simulink model "Sensor_Implementation"  (R2017a)
settings: Solver=VariableStepAuto  StartTime=0.0  StopTime=1000  RelTol=1e-3
libraries: simulink x6
settings Model: Creator=GusBus  LastModifiedBy=GusBus

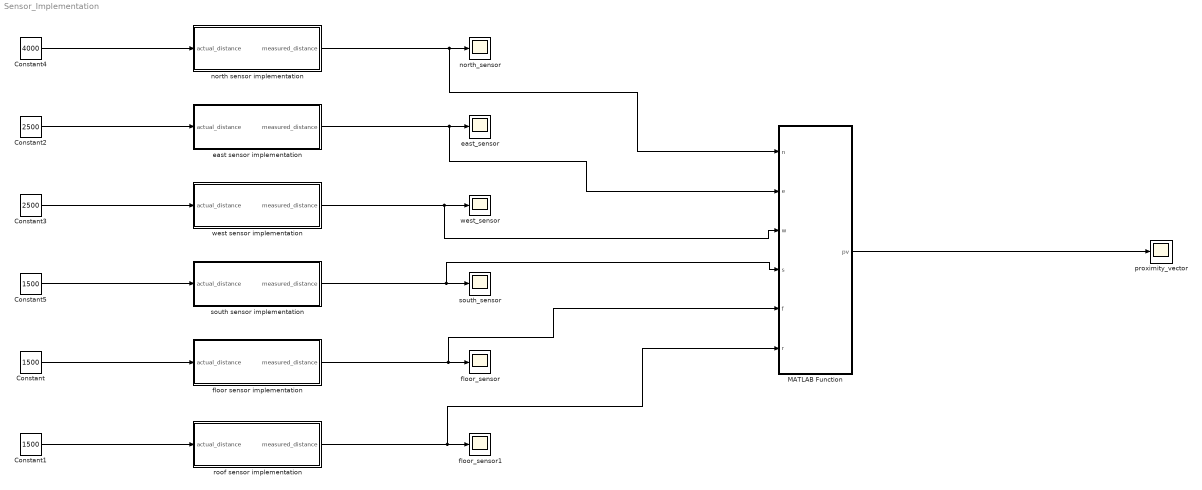
== system Sensor_Implementation ==
  Constant : Constant  Value=1500
  Constant1 : Constant  Value=1500
  Constant2 : Constant  Value=2500
  Constant3 : Constant  Value=2500
  Constant4 : Constant  Value=4000
  Constant5 : Constant  Value=1500
  MATLAB Function : MATLAB Function  TreatAsAtomicUnit=on
  east sensor implementation : Subsystem
  east_sensor : Scope
  floor sensor implementation : Subsystem
  floor_sensor : Scope
  floor_sensor1 : Scope
  north sensor implementation : Subsystem
  north_sensor : Scope
  proximity_vector : Scope
  roof sensor implementation : Subsystem
  south sensor implementation : Subsystem
  south_sensor : Scope
  west sensor implementation : Subsystem
  west_sensor : Scope
  wires:
  Constant/1 -> floor sensor implementation/1(actual_distance)
  floor sensor implementation/1(measured_distance) -> MATLAB Function/5(f), floor_sensor/1
  roof sensor implementation/1(measured_distance) -> MATLAB Function/6(r), floor_sensor1/1
  Constant1/1 -> roof sensor implementation/1(actual_distance)
  east sensor implementation/1(measured_distance) -> east_sensor/1, MATLAB Function/2(e)
  Constant2/1 -> east sensor implementation/1(actual_distance)
  west sensor implementation/1(measured_distance) -> MATLAB Function/3(w), west_sensor/1
  Constant3/1 -> west sensor implementation/1(actual_distance)
  Constant4/1 -> north sensor implementation/1(actual_distance)
  north sensor implementation/1(measured_distance) -> MATLAB Function/1(n), north_sensor/1
  Constant5/1 -> south sensor implementation/1(actual_distance)
  south sensor implementation/1(measured_distance) -> MATLAB Function/4(s), south_sensor/1
  MATLAB Function/1(pv) -> proximity_vector/1

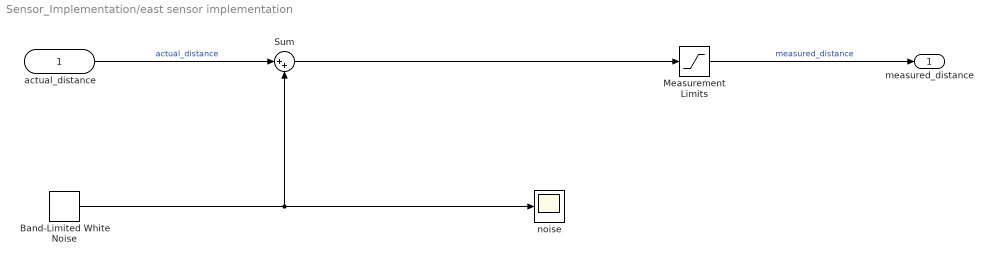
== system Sensor_Implementation/east sensor implementation ==
  actual_distance : Inport
  Band-Limited White Noise : simulink/Sources/Band-Limited White Noise  Cov=[0.01]  Ts=0.1  seed=[23341]
  Measurement Limits : Saturate  UpperLimit=4000  LowerLimit=40
  Sum : Sum  Inputs=|++
  noise : Scope
  measured_distance : Outport
  wires:
  actual_distance/1 -> Sum/1  "actual_distance"
  Measurement Limits/1 -> measured_distance/1  "measured_distance"
  Band-Limited White Noise/1 -> noise/1, Sum/2
  Sum/1 -> Measurement Limits/1

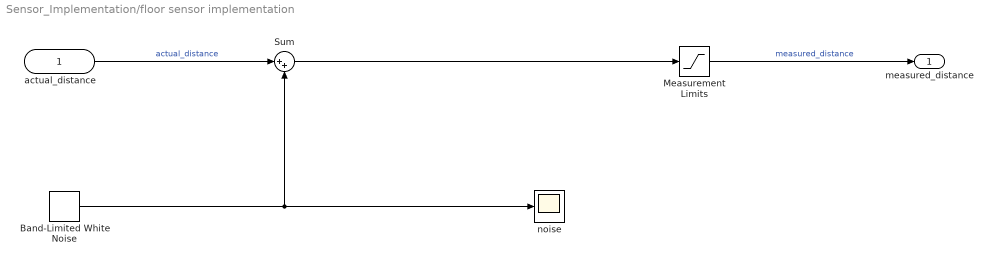
== system Sensor_Implementation/floor sensor implementation ==
  actual_distance : Inport
  Band-Limited White Noise : simulink/Sources/Band-Limited White Noise  Cov=[0.01]  Ts=0.1  seed=[23341]
  Measurement Limits : Saturate  UpperLimit=4000  LowerLimit=40
  Sum : Sum  Inputs=|++
  noise : Scope
  measured_distance : Outport
  wires:
  actual_distance/1 -> Sum/1  "actual_distance"
  Measurement Limits/1 -> measured_distance/1  "measured_distance"
  Band-Limited White Noise/1 -> noise/1, Sum/2
  Sum/1 -> Measurement Limits/1

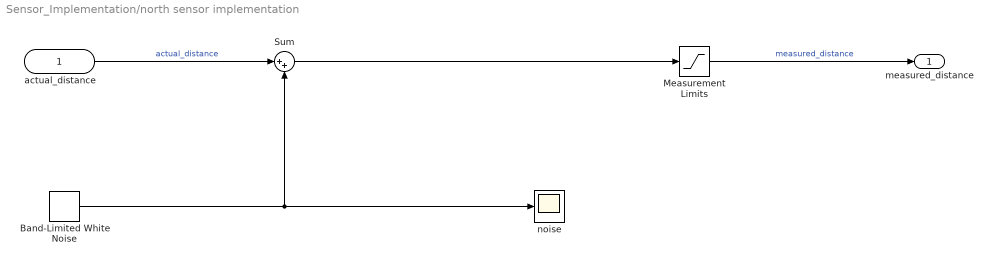
== system Sensor_Implementation/north sensor implementation ==
  actual_distance : Inport
  Band-Limited White Noise : simulink/Sources/Band-Limited White Noise  Cov=[0.01]  Ts=0.1  seed=[23341]
  Measurement Limits : Saturate  UpperLimit=4000  LowerLimit=40
  Sum : Sum  Inputs=|++
  noise : Scope
  measured_distance : Outport
  wires:
  actual_distance/1 -> Sum/1  "actual_distance"
  Measurement Limits/1 -> measured_distance/1  "measured_distance"
  Band-Limited White Noise/1 -> noise/1, Sum/2
  Sum/1 -> Measurement Limits/1

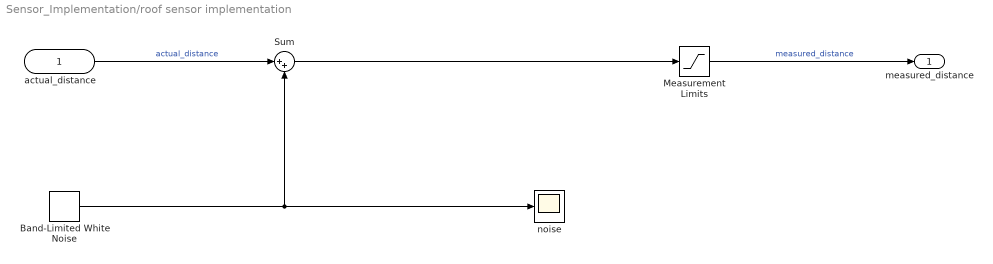
== system Sensor_Implementation/roof sensor implementation ==
  actual_distance : Inport
  Band-Limited White Noise : simulink/Sources/Band-Limited White Noise  Cov=[0.01]  Ts=0.1  seed=[23341]
  Measurement Limits : Saturate  UpperLimit=4000  LowerLimit=40
  Sum : Sum  Inputs=|++
  noise : Scope
  measured_distance : Outport
  wires:
  actual_distance/1 -> Sum/1  "actual_distance"
  Measurement Limits/1 -> measured_distance/1  "measured_distance"
  Band-Limited White Noise/1 -> noise/1, Sum/2
  Sum/1 -> Measurement Limits/1

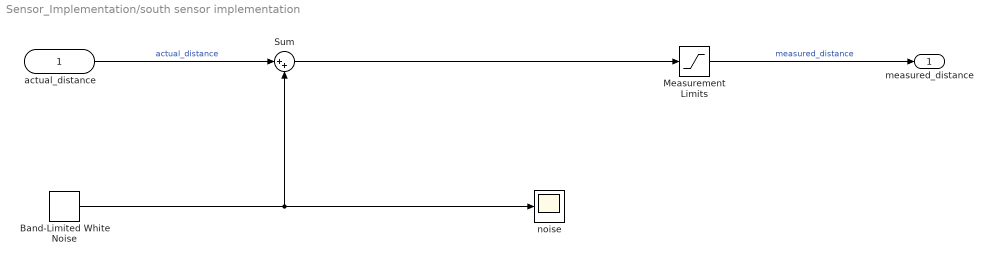
== system Sensor_Implementation/south sensor implementation ==
  actual_distance : Inport
  Band-Limited White Noise : simulink/Sources/Band-Limited White Noise  Cov=[0.01]  Ts=0.1  seed=[23341]
  Measurement Limits : Saturate  UpperLimit=4000  LowerLimit=40
  Sum : Sum  Inputs=|++
  noise : Scope
  measured_distance : Outport
  wires:
  actual_distance/1 -> Sum/1  "actual_distance"
  Measurement Limits/1 -> measured_distance/1  "measured_distance"
  Band-Limited White Noise/1 -> noise/1, Sum/2
  Sum/1 -> Measurement Limits/1

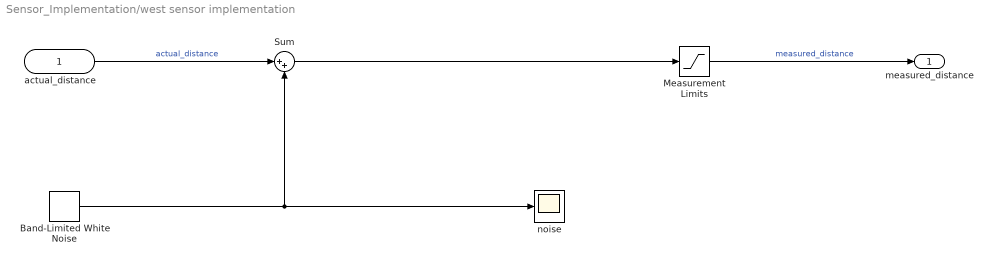
== system Sensor_Implementation/west sensor implementation ==
  actual_distance : Inport
  Band-Limited White Noise : simulink/Sources/Band-Limited White Noise  Cov=[0.01]  Ts=0.1  seed=[23341]
  Measurement Limits : Saturate  UpperLimit=4000  LowerLimit=40
  Sum : Sum  Inputs=|++
  noise : Scope
  measured_distance : Outport
  wires:
  actual_distance/1 -> Sum/1  "actual_distance"
  Measurement Limits/1 -> measured_distance/1  "measured_distance"
  Band-Limited White Noise/1 -> noise/1, Sum/2
  Sum/1 -> Measurement Limits/1

== matlab function Sensor_Implementation/MATLAB Function ==
  data: n input; pv output; e input; w input; s input; f input; r input
function pv = proximityVector(n, e, w, s, f, r)


x = n-s;
y = e-w;
z = f-r;

pv = [x y z];
